simulink model "mySimulink"  (Simulink 7.6)
settings: Solver=ode3  StartTime=0.0  StopTime=inf  FixedStep=1  RelTol=1e-3
PreLoadFcn:
  | init
settings Model: Creator=Frank Poppen  LastModifiedBy=Frank Poppen

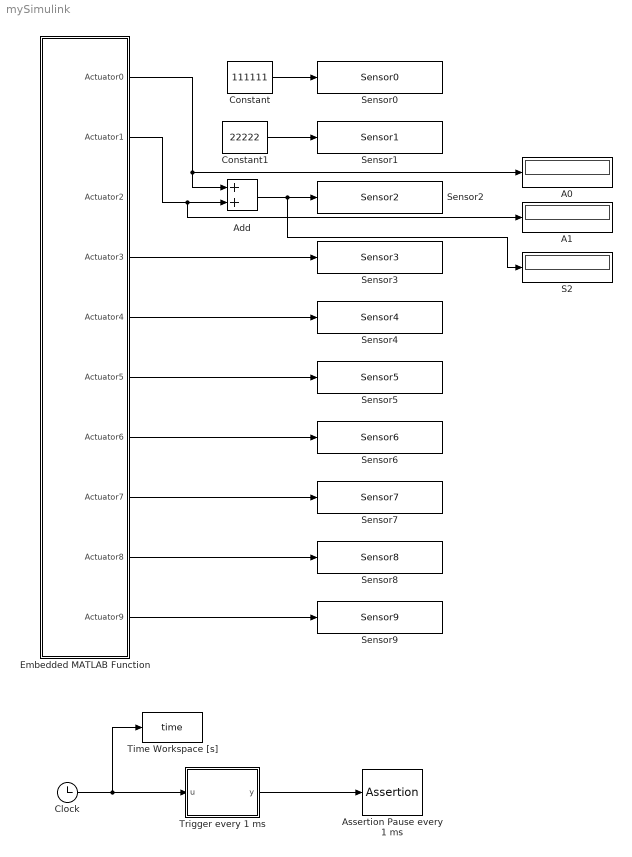
== system mySimulink ==
  A0 : Display
  A1 : Display
  Add : Sum
  Assertion Pause every 1 ms : Assertion  Enabled=on  AssertionFailFcn=set_param(bdroot,'SimulationCommand','pause')  StopWhenAssertionFail=off
  Clock : Clock
      settings: Decimation=10
  Constant : Constant  Value=111111
  Constant1 : Constant  Value=22222
  Embedded MATLAB Function : Stateflow chart  TreatAsAtomicUnit=on
  S2 : Display
  Sensor0 : ToWorkspace  VariableName=Sensor0  SampleTime=-1  SaveFormat=Array
      settings: MaxDataPoints=1
  Sensor1 : ToWorkspace  VariableName=Sensor1  SampleTime=-1  SaveFormat=Array
      settings: MaxDataPoints=1
  Sensor2 : ToWorkspace  VariableName=Sensor2  SampleTime=-1  SaveFormat=Array
      settings: MaxDataPoints=1
  Sensor3 : ToWorkspace  VariableName=Sensor3  SampleTime=-1  SaveFormat=Array
      settings: MaxDataPoints=1
  Sensor4 : ToWorkspace  VariableName=Sensor4  SampleTime=-1  SaveFormat=Array
      settings: MaxDataPoints=1
  Sensor5 : ToWorkspace  VariableName=Sensor5  SampleTime=-1  SaveFormat=Array
      settings: MaxDataPoints=1
  Sensor6 : ToWorkspace  VariableName=Sensor6  SampleTime=-1  SaveFormat=Array
      settings: MaxDataPoints=1
  Sensor7 : ToWorkspace  VariableName=Sensor7  SampleTime=-1  SaveFormat=Array
      settings: MaxDataPoints=1
  Sensor8 : ToWorkspace  VariableName=Sensor8  SampleTime=-1  SaveFormat=Array
      settings: MaxDataPoints=1
  Sensor9 : ToWorkspace  VariableName=Sensor9  SampleTime=-1  SaveFormat=Array
      settings: MaxDataPoints=1
  Time Workspace [s] : ToWorkspace  VariableName=time  SampleTime=-1  SaveFormat=Array
      settings: MaxDataPoints=1
  Trigger every 1 ms : Stateflow chart  TreatAsAtomicUnit=on
  wires:
  Embedded MATLAB Function/1(Actuator0) -> Add/1, A0/1
  Embedded MATLAB Function/2(Actuator1) -> Add/2, A1/1
  Embedded MATLAB Function/4(Actuator3) -> Sensor3/1
  Embedded MATLAB Function/5(Actuator4) -> Sensor4/1
  Embedded MATLAB Function/6(Actuator5) -> Sensor5/1
  Embedded MATLAB Function/7(Actuator6) -> Sensor6/1
  Embedded MATLAB Function/8(Actuator7) -> Sensor7/1
  Embedded MATLAB Function/9(Actuator8) -> Sensor8/1
  Embedded MATLAB Function/10(Actuator9) -> Sensor9/1
  Add/1 -> Sensor2/1, S2/1
  Constant/1 -> Sensor0/1
  Constant1/1 -> Sensor1/1
  Clock/1 -> Time Workspace [s]/1, Trigger every 1 ms/1(u)
  Trigger every 1 ms/1(y) -> Assertion Pause every 1 ms/1

== matlab function Trigger every 1 ms ==
  data: u input double; y output double
function y = fcn(u)
%#eml

% The modulo function defines the time steps after which the
% simulation is paused, after continued by SystemC model. Even
% though mathworks interprets time in 1 seconds we just reinterpret
% 1 time unit as 1 minute.
% We want to sync our two simulations (Simulink & SystemC) with 0.017 Hz.
% So we devide by 1 minute to stop after each minute of time. 

y = mod(u,1);

== matlab function Embedded MATLAB Function ==
  data: Actuator0 output double; Actuator1 output double; Actuator2 output double; Actuator3 output double; Actuator4 output double; Actuator5 output double; Actuator6 output double; Actuator7 output double; Actuator8 output double; Actuator9 output double
function [Actuator0, Actuator1, Actuator2, Actuator3, Actuator4, Actuator5, Actuator6, Actuator7, Actuator8, Actuator9] = actuatorRead()
%#eml

eml.extrinsic('evalin');
eml.extrinsic('assignin');

% If we do not initialize values in this way, Actuators would be
% created during first assignment below and inherit the type 'MATLAB TYPE'
% But this is not a valid type for a function output. could not figure out
% a quick way do fix this with typecast or similar. This initialization is
% a workaround that works (even though it is not nice).
Actuator0 = 0.0;
Actuator1 = 0.0;
Actuator2 = 0.0;
Actuator3 = 0.0;
Actuator4 = 0.0;
Actuator5 = 0.0;
Actuator6 = 0.0;
Actuator7 = 0.0;
Actuator8 = 0.0;
Actuator9 = 0.0;

% The actuator(i) variables in the matlab workspace are created and initialised in the init.m file
% which is executed just before the start of the model. Make sure that in
% that init.m file you have the number of actuators you are going to use
% here specified.
% Be aware that in C we start counting at '0' while matlab arrays start
% counting at '1'
Actuator0 = evalin('base','Actuator0');
Actuator1 = evalin('base','Actuator1');
Actuator2 = evalin('base','Actuator2');
Actuator3 = evalin('base','Actuator3');
Actuator4 = evalin('base','Actuator4');
Actuator5 = evalin('base','Actuator5');
Actuator6 = evalin('base','Actuator6');
Actuator7 = evalin('base','Actuator7');
Actuator8 = evalin('base','Actuator8');
Actuator9 = evalin('base','Actuator9');
